simulink model "full_model_steady_state"  (R2017b)
settings: Solver=ode1  StartTime=0.0  StopTime=100  FixedStep=0.001  RelTol=1e-3
undefined symbols (not defined in the file): pars
settings Model: Creator=michaelchadwick  LastModifiedBy=emiel

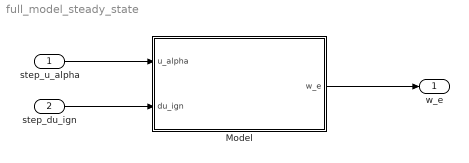
== system full_model_steady_state ==
  step_u_alpha : Inport
  step_du_ign : Inport  Port=2
  Model : Subsystem
  w_e : Outport
  wires:
  Model/1(w_e) -> w_e/1
  step_u_alpha/1 -> Model/1(u_alpha)
  step_du_ign/1 -> Model/2(du_ign)

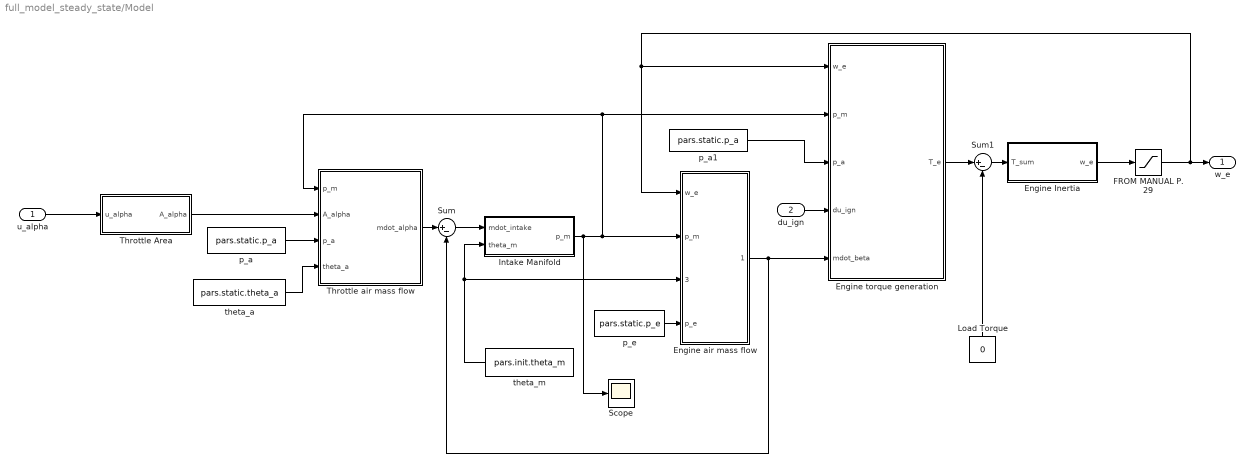
== system full_model_steady_state/Model ==
  u_alpha : Inport
  du_ign : Inport  Port=2
  Engine Inertia : Subsystem
  Engine air mass flow : Subsystem
  Engine torque generation : Subsystem
  "FROM MANUAL P. 29 " : Saturate  UpperLimit=500  LowerLimit=20
  Intake Manifold : Subsystem
  Load Torque : Constant  Value=0
  Scope : Scope
  Sum : Sum  Inputs=|+-
  Sum1 : Sum  Inputs=|+-
  Throttle Area : Subsystem
  Throttle air mass flow : Subsystem
  p_a : Constant  Value=pars.static.p_a
  p_a1 : Constant  Value=pars.static.p_a
  p_e : Constant  Value=pars.static.p_e
  theta_a : Constant  Value=pars.static.theta_a
  theta_m : Constant  Value=pars.init.theta_m
  w_e : Outport
  wires:
  Sum/1 -> Intake Manifold/1(mdot_intake)
  du_ign/1 -> Engine torque generation/4(du_ign)
  theta_a/1 -> Throttle air mass flow/4(theta_a)
  Intake Manifold/1(p_m) -> Throttle air mass flow/1(p_m), Engine torque generation/2(p_m), Engine air mass flow/2(p_m), Scope/1
  theta_m/1 -> Intake Manifold/2(theta_m), Engine air mass flow/3(theta_m)
  p_a1/1 -> Engine torque generation/3(p_a)
  p_a/1 -> Throttle air mass flow/3(p_a)
  Throttle Area/1(A_alpha) -> Throttle air mass flow/2(A_alpha)
  Engine air mass flow/1(mdot_beta) -> Sum/2, Engine torque generation/5(mdot_beta)
  Sum1/1 -> Engine Inertia/1(T_sum)
  Engine torque generation/1(T_e) -> Sum1/1
  u_alpha/1 -> Throttle Area/1(u_alpha)
  p_e/1 -> Engine air mass flow/4(p_e)
  Engine Inertia/1(w_e) -> "FROM MANUAL P. 29 "/1
  Throttle air mass flow/1(mdot_alpha) -> Sum/1
  "FROM MANUAL P. 29 "/1 -> Engine torque generation/1(w_e), Engine air mass flow/1(w_e), w_e/1
  Load Torque/1 -> Sum1/2

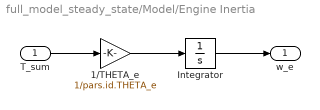
== system full_model_steady_state/Model/Engine Inertia ==
  T_sum : Inport
  1/THETA_e : Gain  Gain=1/pars.id.THETA_e
  Integrator : Integrator  InitialCondition=pars.init.w_e
  w_e : Outport
  wires:
  1/THETA_e/1 -> Integrator/1
  Integrator/1 -> w_e/1
  T_sum/1 -> 1/THETA_e/1

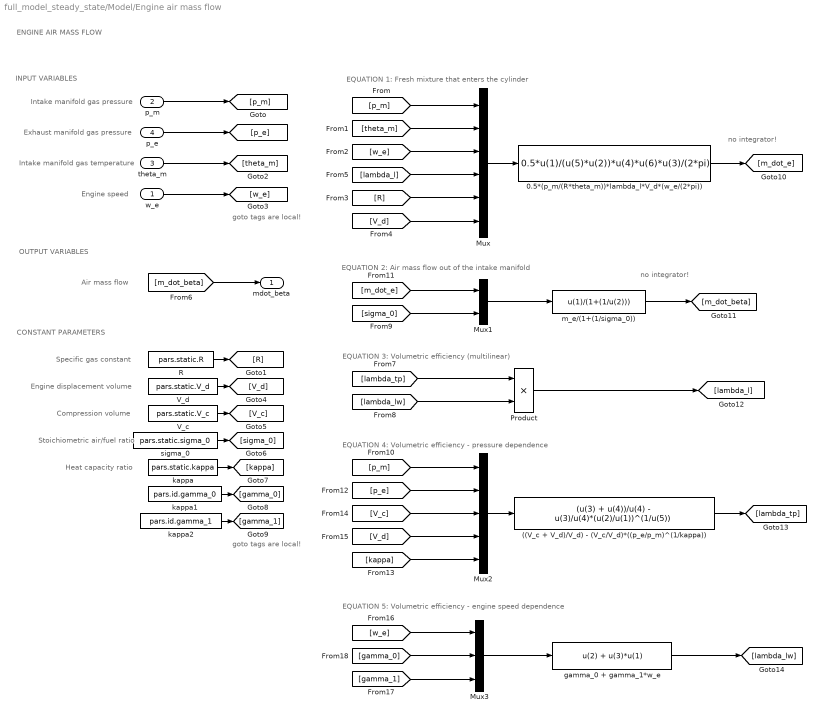
== system full_model_steady_state/Model/Engine air mass flow ==
  note: Specific gas constant
  note: Air mass flow
  note: no integrator!
  note: goto tags are local!
  note: CONSTANT PARAMETERS
  note: Stoichiometric air/fuel ratio
  note: INPUT VARIABLES
  note: EQUATION 4: Volumetric efficiency - pressure dependence
  note: Heat capacity ratio
  note: EQUATION 1: Fresh mixture that enters the cylinder
  note: EQUATION 2: Air mass flow out of the intake manifold
  note: goto tags are local!
  note: ENGINE AIR MASS FLOW
  note: no integrator!
  note: EQUATION 5: Volumetric efficiency - engine speed dependence
  note: Intake manifold gas pressure
  note: Exhaust manifold gas pressure
  note: EQUATION 3: Volumetric efficiency (multilinear)
  note: Intake manifold gas temperature
  note: Compression volume
  note: Engine speed
  note: OUTPUT VARIABLES
  note: Engine displacement volume
  w_e : Inport
  p_m : Inport  Port=2
  theta_m : Inport  Port=3
  p_e : Inport  Port=4
  ((V_c + V_d)/V_d) - (V_c/V_d)*((p_e/p_m)^(1/kappa)) : Fcn  Expr=(u(3) + u(4))/u(4) - u(3)/u(4)*(u(2)/u(1))^(1/u(5))
  0.5*(p_m/(R*theta_m))*lambda_l*V_d*(w_e/(2*pi)) : Fcn  Expr=0.5*u(1)/(u(5)*u(2))*u(4)*u(6)*u(3)/(2*pi)
  Mux : Mux  Inputs=6
  Mux1 : Mux  Inputs=2
  Mux2 : Mux  Inputs=5
  Mux3 : Mux  Inputs=3
  Product : Product
  R : Constant  Value=pars.static.R
  V_c : Constant  Value=pars.static.V_c
  V_d : Constant  Value=pars.static.V_d
  gamma_0 + gamma_1*w_e : Fcn  Expr=u(2) + u(3)*u(1)
  kappa : Constant  Value=pars.static.kappa
  kappa1 : Constant  Value=pars.id.gamma_0
  kappa2 : Constant  Value=pars.id.gamma_1
  m_e/(1+(1/sigma_0)) : Fcn  Expr=u(1)/(1+(1/u(2)))
  sigma_0 : Constant  Value=pars.static.sigma_0
  mdot_beta : Outport
  wires:
  kappa/1 -> [kappa]
  [m_dot_beta] -> mdot_beta/1
  [V_d] -> Mux2/4
  [gamma_0] -> Mux3/2
  [w_e] -> Mux3/1
  [p_m] -> Mux2/1
  Mux2/1 -> ((V_c + V_d)/V_d) - (V_c/V_d)*((p_e/p_m)^(1/kappa))/1
  kappa1/1 -> [gamma_0]
  ((V_c + V_d)/V_d) - (V_c/V_d)*((p_e/p_m)^(1/kappa))/1 -> [lambda_tp]
  m_e/(1+(1/sigma_0))/1 -> [m_dot_beta]
  [gamma_1] -> Mux3/3
  w_e/1 -> [w_e]
  Mux3/1 -> gamma_0 + gamma_1*w_e/1
  Mux/1 -> 0.5*(p_m/(R*theta_m))*lambda_l*V_d*(w_e/(2*pi))/1
  [p_m] -> Mux/1
  [m_dot_e] -> Mux1/1
  [V_c] -> Mux2/3
  Product/1 -> [lambda_l]
  p_m/1 -> [p_m]
  [lambda_tp] -> Product/1
  [lambda_l] -> Mux/4
  [R] -> Mux/5
  [lambda_lw] -> Product/2
  [w_e] -> Mux/3
  [V_d] -> Mux/6
  sigma_0/1 -> [sigma_0]
  [theta_m] -> Mux/2
  [sigma_0] -> Mux1/2
  kappa2/1 -> [gamma_1]
  Mux1/1 -> m_e/(1+(1/sigma_0))/1
  p_e/1 -> [p_e]
  V_d/1 -> [V_d]
  [p_e] -> Mux2/2
  gamma_0 + gamma_1*w_e/1 -> [lambda_lw]
  [kappa] -> Mux2/5
  R/1 -> [R]
  V_c/1 -> [V_c]
  0.5*(p_m/(R*theta_m))*lambda_l*V_d*(w_e/(2*pi))/1 -> [m_dot_e]
  theta_m/1 -> [theta_m]

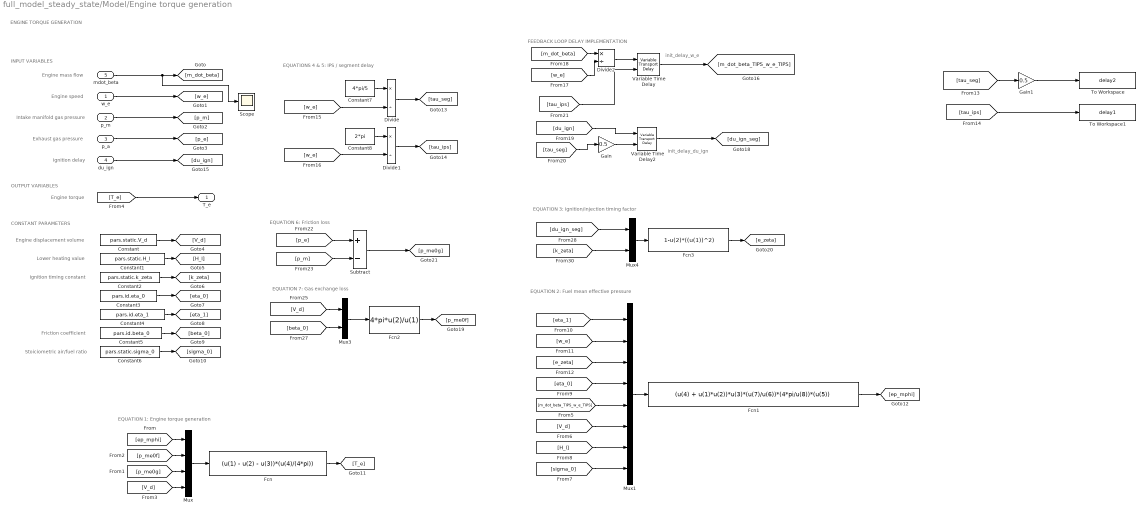
== system full_model_steady_state/Model/Engine torque generation ==
  note: Engine speed
  note: CONSTANT PARAMETERS
  note: Engine mass flow
  note: Exhaust gas pressure
  note: Engine torque
  note: ENGINE TORQUE GENERATION
  note: Friction coefficient
  note: EQUATION 2: Fuel mean effective pressure
  note: init_delay_w_e
  note: INPUT VARIABLES
  note: EQUATION 7: Gas exchange loss
  note: Ignition delay
  note: init_delay_du_ign
  note: Stoiciometric air/fuel ratio
  note: Ignition timing constant
  note: OUTPUT VARIABLES
  note: EQUATION 3: Ignition/injection timing factor
  note: EQUATION 1: Engine torque generation
  note: EQUATION 6: Friction loss
  note: Engine displacement volume
  note: Intake manifold gas pressure
  note: Lower heating value
  note: FEEDBACK LOOP DELAY IMPLEMENTATION
  note: EQUATIONS 4 & 5: IPS / segment delay
  w_e : Inport
  p_m : Inport  Port=2
  p_a : Inport  Port=3
  du_ign : Inport  Port=4
  mdot_beta : Inport  Port=5
  Constant : Constant  Value=pars.static.V_d
  Constant1 : Constant  Value=pars.static.H_l
  Constant2 : Constant  Value=pars.static.k_zeta
  Constant3 : Constant  Value=pars.id.eta_0
  Constant4 : Constant  Value=pars.id.eta_1
  Constant5 : Constant  Value=pars.id.beta_0
  Constant6 : Constant  Value=pars.static.sigma_0
  Constant7 : Constant  Value=4*pi/5
  Constant8 : Constant  Value=2*pi
  Divide : Product  Inputs=*/
  Divide1 : Product  Inputs=*/
  Divide2 : Product  Inputs=*/
  Fcn : Fcn  Expr=(u(1) - u(2) - u(3))*(u(4)/(4*pi))
  Fcn1 : Fcn  Expr=(u(4) + u(1)*u(2))*u(3)*(u(7)/u(6))*(4*pi/u(8))*(u(5))
  Fcn2 : Fcn  Expr=4*pi*u(2)/u(1)
  Fcn3 : Fcn  Expr=1-u(2)*((u(1))^2)
  Gain : Gain  Gain=0.5
  Gain1 : Gain  Gain=0.5
  Mux : Mux
  Mux1 : Mux  Inputs=8
  Mux3 : Mux  Inputs=2
  Mux4 : Mux  Inputs=2
  Scope : Scope
  Subtract : Sum  Inputs=+-
  To Workspace : ToWorkspace  VariableName=delay2  SaveFormat=Timeseries  SampleTime=-1
  To Workspace1 : ToWorkspace  VariableName=delay1  SaveFormat=Timeseries  SampleTime=-1
  Variable Time Delay : VariableTransportDelay  MaximumDelay=10  InitialOutput=pars.init.delay_m_dot_beta/pars.init.delay_w_e  MaximumPoints=10240
  Variable Time Delay2 : VariableTransportDelay  MaximumDelay=10  InitialOutput=pars.init.delay_du_ign  MaximumPoints=10240
  T_e : Outport
  wires:
  Mux1/1 -> Fcn1/1
  Fcn3/1 -> [e_zeta]
  p_a/1 -> [p_e]
  [p_m] -> Subtract/2
  Mux/1 -> Fcn/1
  [du_ign] -> Variable Time Delay2/1
  Mux4/1 -> Fcn3/1
  du_ign/1 -> [du_ign]
  Divide2/1 -> Variable Time Delay/1
  Variable Time Delay/1 -> [m_dot_beta_TIPS_w_e_TIPS]
  Mux3/1 -> Fcn2/1
  Fcn2/1 -> [p_me0f]
  [tau_seg] -> Gain/1
  [ep_mphi] -> Mux/1
  Divide/1 -> [tau_seg]
  [V_d] -> Mux3/1
  Subtract/1 -> [p_me0g]
  [e_zeta] -> Mux1/3
  p_m/1 -> [p_m]
  [eta_0] -> Mux1/4
  [beta_0] -> Mux3/2
  [w_e] -> Divide/2
  Divide1/1 -> [tau_ips]
  [eta_1] -> Mux1/1
  [H_l] -> Mux1/7
  Gain/1 -> Variable Time Delay2/2
  Constant6/1 -> [sigma_0]
  Constant7/1 -> Divide/1
  [p_e] -> Subtract/1
  Constant4/1 -> [eta_1]
  [sigma_0] -> Mux1/8
  [k_zeta] -> Mux4/2
  [V_d] -> Mux1/6
  Fcn/1 -> [T_e]
  Constant8/1 -> Divide1/1
  [du_ign_seg] -> Mux4/1
  Constant1/1 -> [H_l]
  [w_e] -> Mux1/2
  [V_d] -> Mux/4
  [p_me0f] -> Mux/2
  Variable Time Delay2/1 -> [du_ign_seg]
  [T_e] -> T_e/1
  [p_me0g] -> Mux/3
  Constant3/1 -> [eta_0]
  Constant/1 -> [V_d]
  Fcn1/1 -> [ep_mphi]
  mdot_beta/1 -> Scope/1, [m_dot_beta]
  Constant2/1 -> [k_zeta]
  Constant5/1 -> [beta_0]
  w_e/1 -> [w_e]
  [w_e] -> Divide1/2
  [m_dot_beta_TIPS_w_e_TIPS] -> Mux1/5
  [m_dot_beta] -> Divide2/1
  [w_e] -> Divide2/2
  [tau_ips] -> Variable Time Delay/2
  [tau_seg] -> Gain1/1
  [tau_ips] -> To Workspace1/1
  Gain1/1 -> To Workspace/1

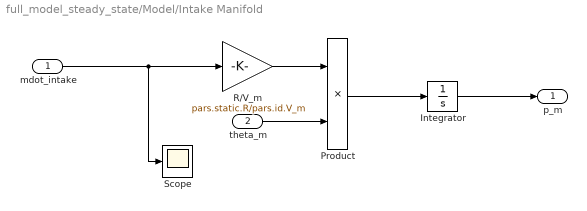
== system full_model_steady_state/Model/Intake Manifold ==
  mdot_intake : Inport
  theta_m : Inport  Port=2
  Integrator : Integrator  InitialCondition=pars.init.p_m
  Product : Product
  R/V_m : Gain  Gain=pars.static.R/pars.id.V_m
  Scope : Scope
  p_m : Outport
  wires:
  R/V_m/1 -> Product/1
  theta_m/1 -> Product/2
  Product/1 -> Integrator/1
  Integrator/1 -> p_m/1
  mdot_intake/1 -> R/V_m/1, Scope/1

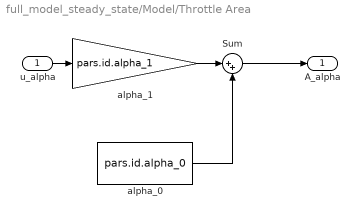
== system full_model_steady_state/Model/Throttle Area ==
  u_alpha : Inport
  Sum : Sum  Inputs=|++
  alpha_0 : Constant  Value=pars.id.alpha_0
  alpha_1 : Gain  Gain=pars.id.alpha_1
  A_alpha : Outport
  wires:
  u_alpha/1 -> alpha_1/1
  alpha_0/1 -> Sum/2
  alpha_1/1 -> Sum/1
  Sum/1 -> A_alpha/1

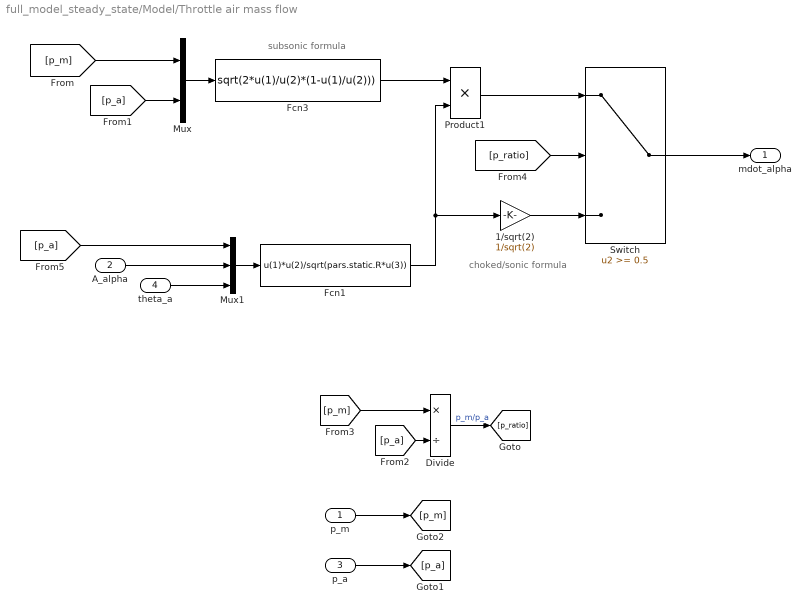
== system full_model_steady_state/Model/Throttle air mass flow ==
  note: choked/sonic formula
  note: subsonic formula
  p_m : Inport
  A_alpha : Inport  Port=2
  p_a : Inport  Port=3
  theta_a : Inport  Port=4
  1/sqrt(2) : Gain  Gain=1/sqrt(2)
  Divide : Product  Inputs=*/
  Fcn1 : Fcn  Expr=u(1)*u(2)/sqrt(pars.static.R*u(3))
  Fcn3 : Fcn  Expr=sqrt(2*u(1)/u(2)*(1-u(1)/u(2)))
  Mux : Mux  Inputs=2
  Mux1 : Mux  Inputs=3
  Product1 : Product
  Switch : Switch  Threshold=0.5
  mdot_alpha : Outport
  wires:
  A_alpha/1 -> Mux1/2
  theta_a/1 -> Mux1/3
  Fcn1/1 -> Product1/2, 1/sqrt(2)/1
  Mux/1 -> Fcn3/1
  Switch/1 -> mdot_alpha/1
  Fcn3/1 -> Product1/1
  Mux1/1 -> Fcn1/1
  Divide/1 -> [p_ratio]  "p_m/p_a"
  p_m/1 -> [p_m]
  p_a/1 -> [p_a]
  [p_m] -> Mux/1
  [p_a] -> Mux/2
  [p_a] -> Divide/2
  [p_m] -> Divide/1
  [p_ratio] -> Switch/2
  [p_a] -> Mux1/1
  Product1/1 -> Switch/1
  1/sqrt(2)/1 -> Switch/3
